simulink model "CLIK_G18"  (R2016a)
settings: Solver=VariableStepAuto  StartTime=0.0  StopTime=20  RelTol=1e-3
libraries: vrlib x7, simulink_extras x6, dspinverses x1
settings Model: Creator=Catarina  LastModifiedBy=Catarina

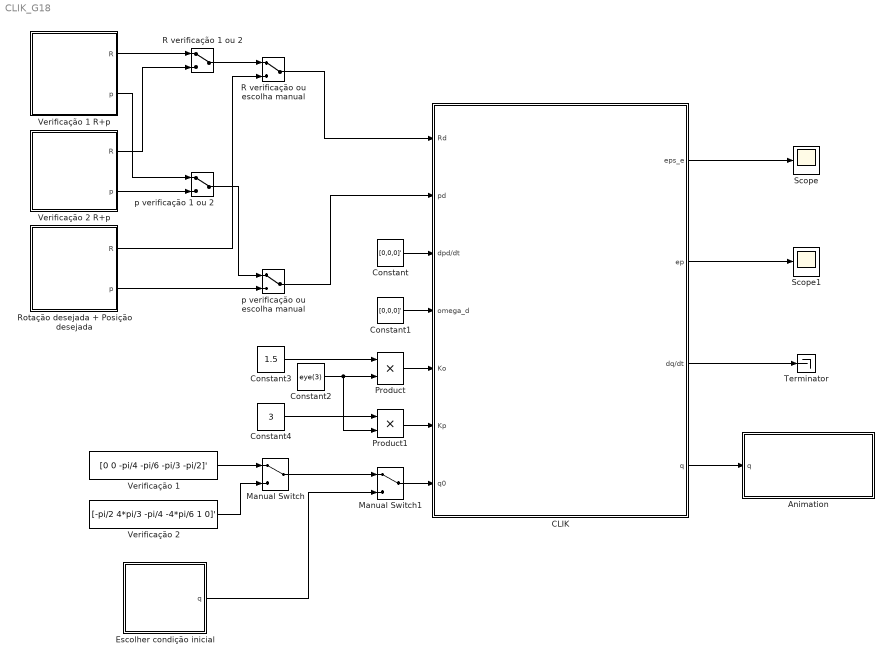
== system CLIK_G18 ==
  "Animation " : Subsystem
  CLIK : Subsystem
  Constant : Constant  Value=[0,0,0]'  VectorParams1D=off
  Constant1 : Constant  Value=[0,0,0]'  VectorParams1D=off
  Constant2 : Constant  Value=eye(3)
  Constant3 : Constant  Value=1.5
  Constant4 : Constant  Value=3
  "Escolher condição inicial " : Subsystem  mask{q1=0, q2=0, q3=0, q4=0, q5=0, q6=0}
  Manual Switch : ManualSwitch
  Manual Switch1 : ManualSwitch
  Product : Product
  Product1 : Product
  R verificação 1 ou 2 : ManualSwitch
  R verificação ou escolha manual : ManualSwitch
  Rotação desejada + Posição desejada : Subsystem  mask{px=0.663, py=-0.109, pz=0.051, phi=0, theta=-180.0, psi=90}
  Scope : Scope
  Scope1 : Scope
  Terminator : Terminator
  Verificação 1 : Constant  Value=[0 0 -pi/4 -pi/6 -pi/3 -pi/2]'  VectorParams1D=off
  Verificação 1 R+p : Subsystem
  Verificação 2 : Constant  Value=[-pi/2 4*pi/3 -pi/4 -4*pi/6 1 0]'  VectorParams1D=off
  Verificação 2 R+p : Subsystem
  p verificação 1 ou 2 : ManualSwitch
  p verificação ou escolha manual : ManualSwitch
  wires:
  CLIK/2(ep) -> Scope1/1
  CLIK/1(eps_e) -> Scope/1
  CLIK/4(q) -> "Animation "/1("q ")
  Constant/1 -> CLIK/3(dpd/dt)
  CLIK/3(dq/dt) -> Terminator/1
  Constant1/1 -> CLIK/4(omega_d)
  Verificação 2/1 -> Manual Switch/2
  Manual Switch1/1 -> CLIK/7(q0)
  Manual Switch/1 -> Manual Switch1/1
  "Escolher condição inicial "/1("q ") -> Manual Switch1/2
  Product/1 -> CLIK/5(Ko)
  Product1/1 -> CLIK/6(Kp)
  Constant2/1 -> Product1/2, Product/2
  Constant3/1 -> Product/1
  Constant4/1 -> Product1/1
  Verificação 1/1 -> Manual Switch/1
  R verificação ou escolha manual/1 -> CLIK/1(Rd)
  p verificação ou escolha manual/1 -> CLIK/2(pd)
  R verificação 1 ou 2/1 -> R verificação ou escolha manual/1
  p verificação 1 ou 2/1 -> p verificação ou escolha manual/1
  Rotação desejada + Posição desejada/1(R) -> R verificação ou escolha manual/2
  Rotação desejada + Posição desejada/2(p) -> p verificação ou escolha manual/2
  Verificação 1 R+p/1(R) -> R verificação 1 ou 2/1
  Verificação 2 R+p/1(R) -> R verificação 1 ou 2/2
  Verificação 2 R+p/2(p) -> p verificação 1 ou 2/2
  Verificação 1 R+p/2(p) -> p verificação 1 ou 2/1

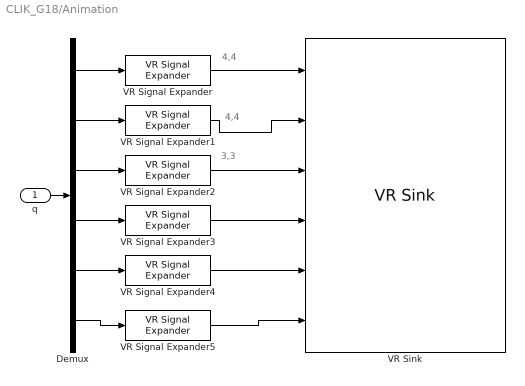
== system CLIK_G18/Animation  ==
  note: 4,4
  note: 3,3
  note: 4,4
  "q " : Inport
  Demux : Demux  Outputs=6
  VR Signal Expander{,1..5} (6 alike) : vrlib/VR Signal Expander  outwidth=4  outidx=4
  VR Sink : vrlib/VR Sink  InstantiateOnLoad=on  SampleTime=0.1  ViewEnable=on  RemoteChange=off  RemoteView=off  FieldsWritten=Jt1_DH_dv.rotation.4.1.1.double#Jt2_DH_dv.rotation.4.1.1.double#Jt3_DH_dv.rotation.4.1.1.double#Jt4_DH_dv.rotation.4.1.1.double#Jt5_DH_dv.rotation.4.1.1.double#Jt6_DH_dv.rotation.4.1.1.double  WorldFileName=RobotG18_Opt_NoAxes.wrl  WorldDescription=D-H Reference Frames for Virtual Reality Robot  AutoView=off  VideoDimensions=[]  AllowVariableSize=off
  wires:
  "q "/1 -> Demux/1
  Demux/1 -> VR Signal Expander/1
  Demux/2 -> VR Signal Expander1/1
  Demux/3 -> VR Signal Expander2/1
  Demux/4 -> VR Signal Expander3/1
  Demux/5 -> VR Signal Expander4/1
  Demux/6 -> VR Signal Expander5/1
  VR Signal Expander/1 -> VR Sink/1
  VR Signal Expander1/1 -> VR Sink/2
  VR Signal Expander5/1 -> VR Sink/6
  VR Signal Expander2/1 -> VR Sink/3
  VR Signal Expander3/1 -> VR Sink/4
  VR Signal Expander4/1 -> VR Sink/5

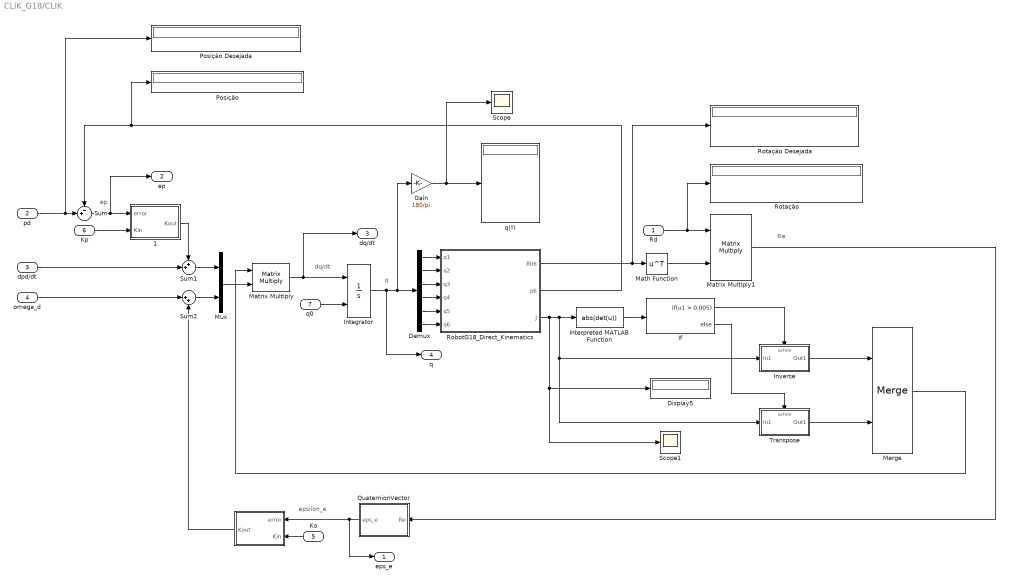
== system CLIK_G18/CLIK ==
  note: epsilon_e
  note: Re
  note: ep
  note: dq/dt
  note: q
  Rd : Inport
  pd : Inport  Port=2
  dpd/dt : Inport  Port=3
  omega_d : Inport  Port=4
  Ko : Inport  Port=5
  Kp : Inport  Port=6
  q0 : Inport  Port=7
  " " : MATLAB Function  TreatAsAtomicUnit=on
  " 1" : MATLAB Function  TreatAsAtomicUnit=on
  Demux : Demux  Outputs=6
  Display5 : Display
  Gain : Gain  Gain=180/pi
  If : If  IfExpression=u1 > 0.005  ZeroCross=off
  Integrator : Integrator  InitialConditionSource=external
  Interpreted MATLAB Function : MATLABFcn  MATLABFcn=abs(det(u))
  Inverse : Subsystem  TreatAsAtomicUnit=on
  Math Function : Math  Operator=transpose  SaturateOnIntegerOverflow=on
  Matrix Multiply : Product  Multiplication=Matrix(*)
  Matrix Multiply1 : Product  Multiplication=Matrix(*)
  Merge : Merge
  Mux : Mux  Inputs=2
  Posição : Display
      settings: Decimation=3
  Posição Desejada : Display
      settings: Decimation=3
  QuaternionVector : MATLAB Function  TreatAsAtomicUnit=on
  RobotG18_Direct_Kinematics : MATLAB Function  TreatAsAtomicUnit=on
  Rotação : Display
      settings: Decimation=3
  Rotação Desejada : Display
      settings: Decimation=3
  Scope : Scope
  Scope1 : Scope
  Sum : Sum  Inputs=-+|
  Sum1 : Sum  Inputs=++|
  Sum2 : Sum  Inputs=|++
  Transpose : Subsystem  TreatAsAtomicUnit=on
  q(º) : Display
  eps_e : Outport
  ep : Outport  Port=2
  dq/dt : Outport  Port=3
  q : Outport  Port=4
  wires:
  Integrator/1 -> q/1, Gain/1, Demux/1
  Demux/3 -> RobotG18_Direct_Kinematics/3(q3)
  Demux/4 -> RobotG18_Direct_Kinematics/4(q4)
  Demux/1 -> RobotG18_Direct_Kinematics/1(q1)
  Demux/2 -> RobotG18_Direct_Kinematics/2(q2)
  Demux/5 -> RobotG18_Direct_Kinematics/5(q5)
  Demux/6 -> RobotG18_Direct_Kinematics/6(q6)
  QuaternionVector/1(eps_e) -> " "/1(error), eps_e/1
  Matrix Multiply/1 -> dq/dt/1, Integrator/1
  Math Function/1 -> Matrix Multiply1/2
  " "/1(Kout) -> Sum2/2
  omega_d/1 -> Sum2/1
  Sum2/1 -> Mux/2
  Sum1/1 -> Mux/1
  Mux/1 -> Matrix Multiply/2
  Rd/1 -> Rotação/1, Matrix Multiply1/1
  Matrix Multiply1/1 -> QuaternionVector/1(Re)
  pd/1 -> Posição Desejada/1, Sum/2
  RobotG18_Direct_Kinematics/2(p6) -> Posição/1, Sum/1
  Sum/1 -> " 1"/1(error), ep/1
  dpd/dt/1 -> Sum1/2
  RobotG18_Direct_Kinematics/1(R06) -> Math Function/1, Rotação Desejada/1
  RobotG18_Direct_Kinematics/3(J) -> Interpreted MATLAB Function/1, Inverse/1(In1), Transpose/1(In1), Display5/1, Scope1/1
  If/1 -> Inverse/Action
  If/2 -> Transpose/Action
  Transpose/1(Out1) -> Merge/2
  Inverse/1(Out1) -> Merge/1
  Merge/1 -> Matrix Multiply/1
  Gain/1 -> Scope/1, q(º)/1
  q0/1 -> Integrator/2
  Ko/1 -> " "/2(Kin)
  " 1"/1(Kout) -> Sum1/1
  Kp/1 -> " 1"/2(Kin)
  Interpreted MATLAB Function/1 -> If/1

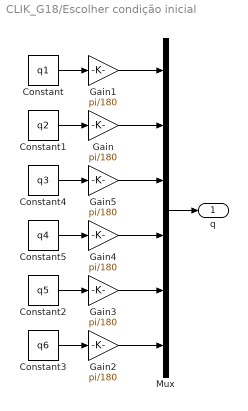
== system CLIK_G18/Escolher condição inicial  ==
  Constant : Constant  Value=q1
  Constant1 : Constant  Value=q2
  Constant2 : Constant  Value=q5
  Constant3 : Constant  Value=q6
  Constant4 : Constant  Value=q3
  Constant5 : Constant  Value=q4
  Gain{,1..5} (6 alike) : Gain  Gain=pi/180
  Mux : Mux  Inputs=6
  "q " : Outport
  wires:
  Constant/1 -> Gain1/1
  Constant1/1 -> Gain/1
  Mux/1 -> "q "/1
  Gain1/1 -> Mux/1
  Gain/1 -> Mux/2
  Constant2/1 -> Gain3/1
  Constant3/1 -> Gain2/1
  Constant4/1 -> Gain5/1
  Constant5/1 -> Gain4/1
  Gain5/1 -> Mux/3
  Gain4/1 -> Mux/4
  Gain3/1 -> Mux/5
  Gain2/1 -> Mux/6

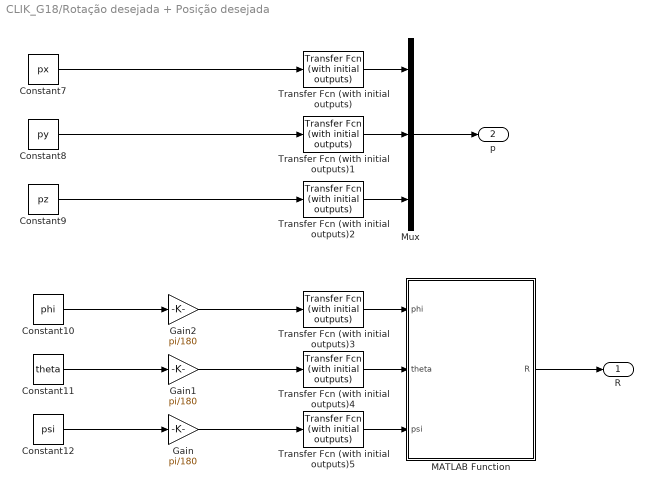
== system CLIK_G18/Rotação desejada + Posição desejada ==
  Constant10 : Constant  Value=phi
  Constant11 : Constant  Value=theta
  Constant12 : Constant  Value=psi
  Constant7 : Constant  Value=px
  Constant8 : Constant  Value=py
  Constant9 : Constant  Value=pz
  Gain : Gain  Gain=pi/180
  Gain1 : Gain  Gain=pi/180
  Gain2 : Gain  Gain=pi/180
  MATLAB Function : MATLAB Function  TreatAsAtomicUnit=on
  Mux : Mux  Inputs=3
  Transfer Fcn (with initial outputs) : simulink_extras/Additional Linear/Transfer Fcn (with initial outputs)  N=[2]  D="[1  2]"  Y0=px  U0=0
  Transfer Fcn (with initial outputs)1 : simulink_extras/Additional Linear/Transfer Fcn (with initial outputs)  N=[2]  D="[1  2]"  Y0=py  U0=0
  Transfer Fcn (with initial outputs)2 : simulink_extras/Additional Linear/Transfer Fcn (with initial outputs)  N=[2]  D="[1  2]"  Y0=pz  U0=0
  Transfer Fcn (with initial outputs)3 : simulink_extras/Additional Linear/Transfer Fcn (with initial outputs)  N=[2]  D="[1  2]"  Y0=phi  U0=0
  Transfer Fcn (with initial outputs)4 : simulink_extras/Additional Linear/Transfer Fcn (with initial outputs)  N=[2]  D="[1  2]"  Y0=theta  U0=0
  Transfer Fcn (with initial outputs)5 : simulink_extras/Additional Linear/Transfer Fcn (with initial outputs)  N=[2]  D="[1  2]"  Y0=psi  U0=0
  R : Outport
  p : Outport  Port=2
  wires:
  Constant8/1 -> Transfer Fcn (with initial outputs)1/1
  Constant9/1 -> Transfer Fcn (with initial outputs)2/1
  Constant12/1 -> Gain/1
  Constant7/1 -> Transfer Fcn (with initial outputs)/1
  Constant11/1 -> Gain1/1
  Constant10/1 -> Gain2/1
  Transfer Fcn (with initial outputs)5/1 -> MATLAB Function/3(psi)
  Transfer Fcn (with initial outputs)3/1 -> MATLAB Function/1(phi)
  Transfer Fcn (with initial outputs)4/1 -> MATLAB Function/2(theta)
  Transfer Fcn (with initial outputs)/1 -> Mux/1
  Transfer Fcn (with initial outputs)1/1 -> Mux/2
  Transfer Fcn (with initial outputs)2/1 -> Mux/3
  Gain2/1 -> Transfer Fcn (with initial outputs)3/1
  Gain1/1 -> Transfer Fcn (with initial outputs)4/1
  Gain/1 -> Transfer Fcn (with initial outputs)5/1
  Mux/1 -> p/1
  MATLAB Function/1(R) -> R/1

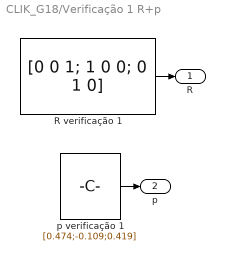
== system CLIK_G18/Verificação 1 R+p ==
  R verificação 1 : Constant  Value=[0 0 1; 1 0 0; 0 1 0]  VectorParams1D=off
  p verificação 1 : Constant  Value=[0.474;-0.109;0.419]  VectorParams1D=off
  R : Outport
  p : Outport  Port=2
  wires:
  p verificação 1/1 -> p/1
  R verificação 1/1 -> R/1

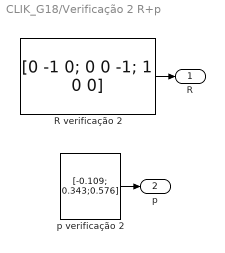
== system CLIK_G18/Verificação 2 R+p ==
  R verificação 2 : Constant  Value=[0 -1 0; 0 0 -1; 1 0 0]  VectorParams1D=off
  p verificação 2 : Constant  Value=[-0.109; 0.343;0.576]  VectorParams1D=off
  R : Outport
  p : Outport  Port=2
  wires:
  p verificação 2/1 -> p/1
  R verificação 2/1 -> R/1

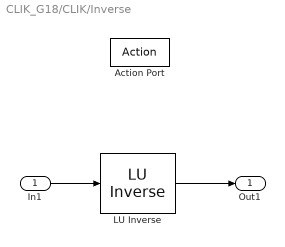
== system CLIK_G18/CLIK/Inverse ==
  In1 : Inport
  Action Port : ActionPort  ActionType=then
  " LU Inverse" : dspinverses/ LU Inverse
  Out1 : Outport
  wires:
  In1/1 -> " LU Inverse"/1
  " LU Inverse"/1 -> Out1/1

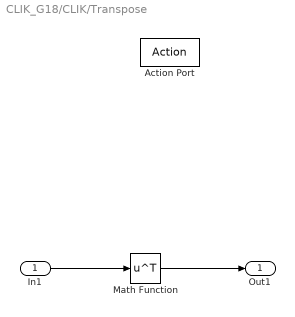
== system CLIK_G18/CLIK/Transpose ==
  In1 : Inport
  Action Port : ActionPort  ActionType=else
  Math Function : Math  Operator=transpose  SaturateOnIntegerOverflow=on
  Out1 : Outport
  wires:
  In1/1 -> Math Function/1
  Math Function/1 -> Out1/1

== matlab function CLIK_G18/CLIK/QuaternionVector ==
  data: Re input; eps_e output
function eps_e  = QuaternionVector(Re)

eps_e = 0.5 * [sign(Re(3,2)-Re(2,3)) * sqrt(abs(Re(1,1)-Re(2,2)-Re(3,3)+1));
               sign(Re(1,3)-Re(3,1)) * sqrt(abs(Re(2,2)-Re(1,1)-Re(3,3)+1));
               sign(Re(2,1)-Re(1,2)) * sqrt(abs(Re(3,3)-Re(1,1)-Re(2,2)+1))];
           
end

== matlab function CLIK_G18/CLIK/RobotG18_Direct_Kinematics ==
  data: q1 input; R06 output; q2 input; q3 input; q4 input; q5 input; q6 input; p6 output; J output
function [R06,p6,J] = RobotG18_Direct_Kinematics(q1,q2,q3,q4,q5,q6)
%#codegen

%    This function was generated by the Symbolic Math Toolbox version 7.0.
%    15-Apr-2021 18:49:51

t2 = q2+q3+q4;
t3 = cos(q1);
t4 = sin(q6);
t5 = sin(q1);
t6 = sin(q5);
t7 = t5.*t6;
t8 = cos(t2);
t9 = cos(q5);
t10 = t7-t3.*t8.*t9;
t11 = sin(t2);
t12 = cos(q6);
t13 = t3.*t6;
t14 = t5.*t8.*t9;
t15 = t13+t14;
t16 = q2+q3;
t17 = cos(q2);
t18 = sin(q2);
t19 = sin(q3);
t20 = cos(t16);
t21 = sin(q4);
t22 = sin(t16);
t23 = cos(q4);
t24 = cos(q3);
t25 = t5.*t17.*(1.7e1./4.0e1);
t26 = t5.*t6.*t8.*(4.1e1./5.0e2);
t27 = t5.*t17.*t24.*(4.9e1./1.25e2);
t28 = t22.*(4.9e1./1.25e2);
t29 = t18.*(1.7e1./4.0e1);
t30 = t20.*t21.*(4.1e1./5.0e2);
t31 = t22.*t23.*(4.1e1./5.0e2);
t32 = t30+t31;
t33 = t6.*t32;
t34 = t20.*t23.*(1.9e1./2.0e2);
t35 = t8.*(1.9e1./2.0e2);
t36 = t6.*t11.*(4.1e1./5.0e2);
t37 = t5.*(1.09e2./1.0e3);
t38 = t3.*t17.*(1.7e1./4.0e1);
t39 = t5.*t9.*(4.1e1./5.0e2);
t40 = t3.*t6.*t8.*(4.1e1./5.0e2);
t41 = t3.*t17.*t24.*(4.9e1./1.25e2);
t42 = t37+t38+t39+t40+t41-t3.*t18.*t19.*(4.9e1./1.25e2)-t3.*t20.*t21.*(1.9e1./2.0e2)-t3.*t22.*t23.*(1.9e1./2.0e2);
t43 = t28+t29+t33+t34-t21.*t22.*(1.9e1./2.0e2);
t44 = t28+t35+t36;
t45 = t35+t36;
t46 = q2+q3+q4+q5;
t47 = sin(t46);
t48 = t47.*(4.1e1./1.0e3);
t49 = t20.*(4.9e1./1.25e2);
t50 = q2+q3+q4-q5;
t51 = sin(t50);
t52 = t5.*t9;
t53 = t3.*t6.*t8;
t54 = t52+t53;
t55 = t5.*t6.*t8;
t56 = t55-t3.*t9;
t57 = t6.*t11;
R06 = reshape([-t10.*t12-t3.*t4.*t11,t12.*t15-t4.*t5.*t11,t4.*t8+t9.*t11.*t12,t4.*t10-t3.*t11.*t12,-t4.*t15-t5.*t11.*t12,t8.*t12-t4.*t9.*t11,t54,t56,t57],[3,3]);
if nargout > 1
    p6 = [t42;t3.*(-1.09e2./1.0e3)+t25+t26+t27-t3.*t9.*(4.1e1./5.0e2)-t5.*t18.*t19.*(4.9e1./1.25e2)-t5.*t20.*t21.*(1.9e1./2.0e2)-t5.*t22.*t23.*(1.9e1./2.0e2);t28+t29+t33+t34-t21.*t22.*(1.9e1./2.0e2)+8.9e1./1.0e3];
end
if nargout > 2
    J = reshape([t3.*(1.09e2./1.0e3)-t25-t26-t27+t3.*t9.*(4.1e1./5.0e2)+t5.*t18.*t19.*(4.9e1./1.25e2)+t5.*t20.*t21.*(1.9e1./2.0e2)+t5.*t22.*t23.*(1.9e1./2.0e2),t42,0.0,0.0,0.0,1.0,-t3.*t43,-t5.*t43,t11.*(-1.9e1./2.0e2)+t17.*(1.7e1./4.0e1)+t48+t49-t51.*(4.1e1./1.0e3),t5,-t3,0.0,-t3.*t44,-t5.*t44,t11.*(-1.9e1./2.0e2)+t48+t49-t51.*(4.1e1./1.0e3),t5,-t3,0.0,-t3.*t45,-t5.*t45,t11.*(-1.9e1./2.0e2)+t48-t51.*(4.1e1./1.0e3),t5,-t3,0.0,t5.*t6.*(-4.1e1./5.0e2)-t3.*t9.*t17.*t19.*t21.*(4.1e1./5.0e2)-t3.*t9.*t18.*t19.*t23.*(4.1e1./5.0e2)-t3.*t9.*t18.*t21.*t24.*(4.1e1./5.0e2)+t3.*t9.*t17.*t23.*t24.*(4.1e1./5.0e2),t3.*t6.*(4.1e1./5.0e2)-t5.*t9.*t17.*t19.*t21.*(4.1e1./5.0e2)-t5.*t9.*t18.*t19.*t23.*(4.1e1./5.0e2)-t5.*t9.*t18.*t21.*t24.*(4.1e1./5.0e2)+t5.*t9.*t17.*t23.*t24.*(4.1e1./5.0e2),t48+t51.*(4.1e1./1.0e3),-t3.*t11,-t5.*t11,t8,0.0,0.0,0.0,t54,t56,t57],[6,6]);
end

== matlab function CLIK_G18/CLIK/  ==
  data: error input; Kin input; Kout output
function Kout = Gains(error, Kin)

Kout = Kin*error;

== matlab function CLIK_G18/Rotação desejada + Posição desejada/MATLAB Function ==
  data: phi input; R output; theta input; psi input
function R  = matriz_R(phi, theta,psi)

s_x = sin(phi);
s_y = sin(theta);
s_z = sin(psi);

c_x = cos(phi);
c_y = cos(theta);
c_z = cos(psi);
 
R = [(c_x*c_y*c_z)-(s_x*s_z)    -(c_x*c_y*s_z)-(s_x*c_z)  c_x*s_y;
     (s_x*c_y*c_z)+(c_x*s_z)    -(s_x*c_y*s_z)+(c_x*c_z)  s_x*s_y;
     -s_y*c_z                    s_y*s_z                  c_y    ];
end

== matlab function CLIK_G18/CLIK/ 1 ==
  data: error input; Kin input; Kout output
function Kout = Gains(error, Kin)

Kout = Kin*error;
